simulink model "simu"  (R2021a)
settings: Solver=VariableStepAuto  StartTime=0.0  StopTime=5  RelTol=1e-3
values from neighbouring files (symbols this model uses):
  Gc = Kp+Ki/s    [clase_code.m]
  Gm = tf(num/den(end),den/den(end))    [clase_code.m]
settings Model: Creator=pierr  LastModifiedBy=pierr

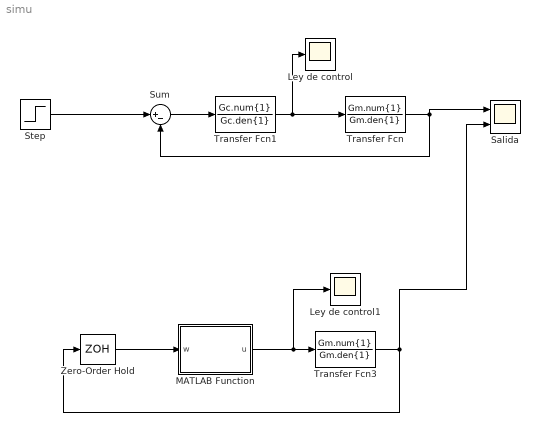
== system simu ==
  Ley de control : Scope
  Ley de control1 : Scope
  MATLAB Function : MATLAB Function  TreatAsAtomicUnit=on
  Salida : Scope  NumInputPorts=2
  Step : Step  Time=0  After=180  SampleTime=0
  Sum : Sum  Inputs=|+-
  Transfer Fcn : TransferFcn  Numerator=Gm.num{1}  Denominator=Gm.den{1}
  Transfer Fcn1 : TransferFcn  Numerator=Gc.num{1}  Denominator=Gc.den{1}
  Transfer Fcn3 : TransferFcn  Numerator=Gm.num{1}  Denominator=Gm.den{1}
  Zero-Order Hold : ZeroOrderHold  SampleTime=0.006
  wires:
  Transfer Fcn1/1 -> Ley de control/1, Transfer Fcn/1
  Sum/1 -> Transfer Fcn1/1
  Transfer Fcn/1 -> Salida/1, Sum/2
  MATLAB Function/1(u) -> Ley de control1/1, Transfer Fcn3/1
  Step/1 -> Sum/1
  Transfer Fcn3/1 -> Zero-Order Hold/1, Salida/2
  Zero-Order Hold/1 -> MATLAB Function/1(w)

== matlab function simu/MATLAB Function ==
  data: w input; u output
function u = fcn(w)
%#codegen
persistent u_1
persistent e_1
if isempty(u_1)
    u_1=0;
    e_1=0;
end

r=450;%establecer referencia

e=r-w;
Ts=0.006;
Kp=0.00727299011414736;
Ki=0.0327284555136631;
u=u_1+(2*Kp+Ki*Ts)/2*e+(Ki*Ts-2*Kp)/2*e_1;
e_1=e;
u_1=u;
